simulink model "Stanley_control"  (R2022b)
settings: Solver=VariableStepAuto  StartTime=0.0  StopTime=60  RelTol=1e-3
values from neighbouring files (symbols this model uses):
  cx = 0:0.1:120    [stanley_ref_01.m]
libraries: Solver_SF x1, simulink x1
settings Model: Creator=admin  LastModifiedBy=admin

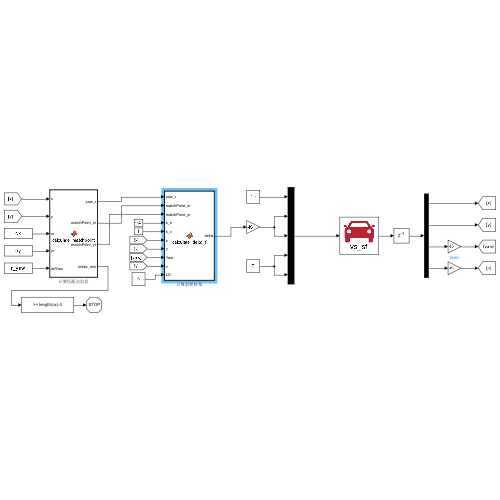
[thumbnail: Simulink's stored preview of the top-level diagram]
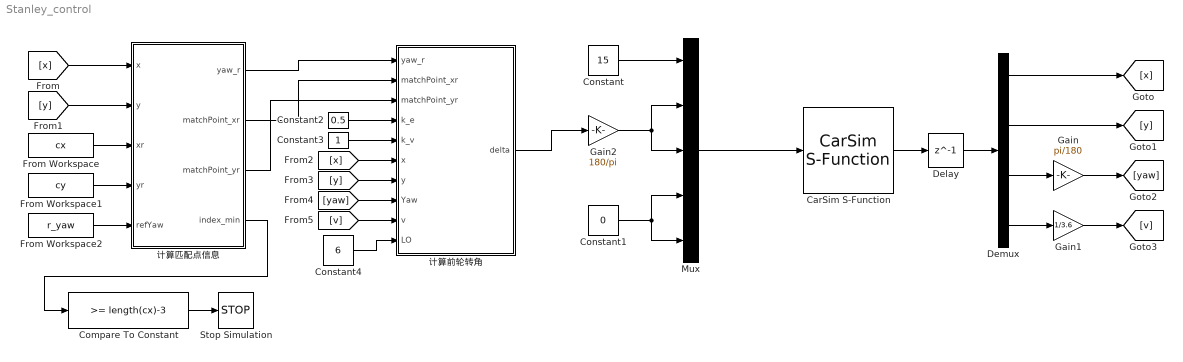
== system Stanley_control ==
  CarSim S-Function : Solver_SF/CarSim S-Function  Priority=1  SIMFILE=simfile.sim  Run_RTs=off  vs_state_ind=Run  StopMode_ind=Vehicle Model
  Compare To Constant : simulink/Logic and Bit Operations/Compare To Constant  relop=>=  const=length(cx)-3  OutDataTypeStr=boolean
  Constant : Constant  Value=15
  Constant1 : Constant  Value=0
  Constant2 : Constant  Value=0.5
  Constant3 : Constant
  Constant4 : Constant  Value=6
  Delay : Delay  DelayLength=1
  Demux : Demux
  From Workspace : FromWorkspace  VariableName=cx
  From Workspace1 : FromWorkspace  VariableName=cy
  From Workspace2 : FromWorkspace  VariableName=r_yaw
  Gain : Gain  Gain=pi/180
  Gain1 : Gain  Gain=1/3.6
  Gain2 : Gain  Gain=180/pi
  Mux : Mux  Inputs=5
  Stop Simulation : Stop
  计算前轮转角 : MATLAB Function  TreatAsAtomicUnit=on
  计算匹配点信息 : MATLAB Function  TreatAsAtomicUnit=on
  wires:
  Demux/1 -> [x]
  Demux/2 -> [y]
  Demux/3 -> Gain/1
  Gain/1 -> [yaw]
  Demux/4 -> Gain1/1
  Gain1/1 -> [v]
  CarSim S-Function/1 -> Delay/1
  Mux/1 -> CarSim S-Function/1
  Constant/1 -> Mux/1
  Gain2/1 -> Mux/3, Mux/2
  Constant1/1 -> Mux/4, Mux/5
  Delay/1 -> Demux/1
  [x] -> 计算匹配点信息/1(x)
  [y] -> 计算匹配点信息/2(y)
  From Workspace/1 -> 计算匹配点信息/3(xr)
  From Workspace1/1 -> 计算匹配点信息/4(yr)
  From Workspace2/1 -> 计算匹配点信息/5(refYaw)
  计算匹配点信息/4(index_min) -> Compare To Constant/1
  Compare To Constant/1 -> Stop Simulation/1
  计算匹配点信息/1(yaw_r) -> 计算前轮转角/1(yaw_r)
  计算匹配点信息/2(matchPoint_xr) -> 计算前轮转角/2(matchPoint_xr)
  计算匹配点信息/3(matchPoint_yr) -> 计算前轮转角/3(matchPoint_yr)
  [x] -> 计算前轮转角/6(x)
  [y] -> 计算前轮转角/7(y)
  [yaw] -> 计算前轮转角/8(Yaw)
  [v] -> 计算前轮转角/9(v)
  Constant2/1 -> 计算前轮转角/4(k_e)
  Constant3/1 -> 计算前轮转角/5(k_v)
  Constant4/1 -> 计算前轮转角/10(LO)
  计算前轮转角/1(delta) -> Gain2/1

== matlab function Stanley_control/计算前轮转角 ==
  data: yaw_r input; delta output; matchPoint_xr input; matchPoint_yr input; k_e input; k_v input; x input; y input; Yaw input; v input; LO input
function delta = calculate_delta_f(yaw_r,matchPoint_xr,matchPoint_yr,k_e,k_v,x,y,Yaw,v,LO)
%*******************CarSim转角向左为正*************************************
    %横向误差：两点距离
    e_y=sqrt((x-matchPoint_xr)^2+(y-matchPoint_yr)^2);

    %判断转向：转换到车辆坐标系下的 纵坐标 正负，小于0，需要向右拐，让其为负值
    dx=x-matchPoint_xr;
    dy=y-matchPoint_yr;
    L_R = dy*cos(Yaw) - dx*sin(Yaw);

    if L_R < 0
       e_y = -e_y;     
    end

    %横向误差产生的控制量
    ey_yaw=atan2(-k_e*e_y,k_v*v+LO);
    %对控制量角度进行限制，使其始终在  -pi到pi之间
    if ey_yaw > pi
        ey_yaw = ey_yaw - 2*pi;
    end
    if ey_yaw < -pi
        ey_yaw = ey_yaw + 2*pi;
    end

    %转角误差：CarSim转角向左为正，自动满足
    ehead_yaw=yaw_r-Yaw;
    %对控制量角度进行限制，使其始终在  -pi到pi之间
    if ehead_yaw > pi
        ehead_yaw = ehead_yaw - 2*pi;
    end
    if ehead_yaw < -pi
        ehead_yaw = ehead_yaw + 2*pi;
    end

    %最两部分组成终前轮转角：
    delta = ehead_yaw+ey_yaw;
    %对最终控制量进行限制，这里假设车辆  向左最多只能转pi/6，向右最多只能转pi/6
    if delta > pi/6
        delta = pi/6;
    end
    if delta < -pi/6
        delta = -pi/6;
    end
end

== matlab function Stanley_control/计算匹配点信息 ==
  data: x input; yaw_r output; y input; xr input; yr input; refYaw input; matchPoint_xr output; matchPoint_yr output; index_min output
function [yaw_r,matchPoint_xr, matchPoint_yr,index_min] = calculate_matchpoint(x,y, xr,yr,refYaw)
    % 找到距离当前位置最近的一个参考轨迹点的序号
    total_point=length(xr);
    distance_min=(x-xr(1))^2+(y-yr(1))^2;
    index_min=1;
    for i = 1:total_point
        d = (x-xr(i))^2+(y-yr(i))^2; 
        if d<distance_min
            distance_min = d;
            index_min=i;
        end
    end

    %通过轨迹点序号得出相关轨迹x,y位置信息与切线夹角
    matchPoint_xr = xr(index_min);
    matchPoint_yr = yr(index_min);
    yaw_r=refYaw(index_min);
end
